simulink model "power_filter"  (R2023b)
settings: Solver=VariableStepAuto  StartTime=0.0  StopTime=.5  RelTol=1e-3
undefined symbols (not defined in the file): T_s, u_gN, w0_pll, w_g
settings Model: Creator=maatt  LastModifiedBy=patet
settings DataIOCC: ReturnWorkspaceOutputs=off

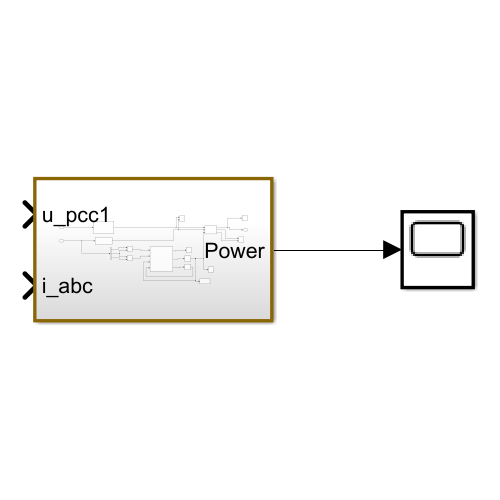
[thumbnail: Simulink's stored preview of the top-level diagram]
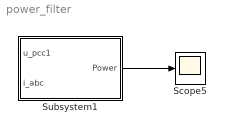
== system power_filter ==
  Scope5 : Scope
  Subsystem1 : Subsystem
  wires:
  Subsystem1/1(Power) -> Scope5/1

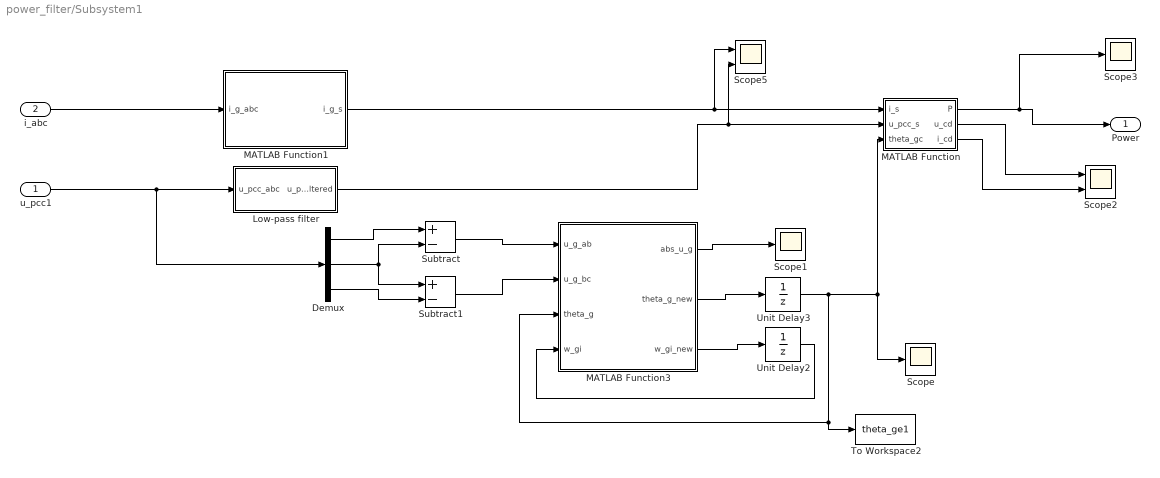
== system power_filter/Subsystem1 ==
  u_pcc1 : Inport
  i_abc : Inport  Port=2
  Demux : Demux  Outputs=3
  Low-pass filter : Subsystem
  MATLAB Function : MATLAB Function  TreatAsAtomicUnit=on
  MATLAB Function1 : MATLAB Function  TreatAsAtomicUnit=on
  MATLAB Function3 : MATLAB Function  TreatAsAtomicUnit=on
  Scope : Scope
  Scope1 : Scope
  Scope2 : Scope  NumInputPorts=2
  Scope3 : Scope
  Scope5 : Scope  NumInputPorts=2
  Subtract : Sum  Inputs=+-
  Subtract1 : Sum  Inputs=+-
  To Workspace2 : ToWorkspace  VariableName=theta_ge1  SaveFormat=Timeseries  SampleTime=-1
  Unit Delay2 : UnitDelay  InitialCondition=w_g  SampleTime=-1  HasFrameUpgradeWarning=on
  Unit Delay3 : UnitDelay  SampleTime=-1  HasFrameUpgradeWarning=on
  Power : Outport
  wires:
  MATLAB Function/1(P) -> Scope3/1, Power/1
  i_abc/1 -> MATLAB Function1/1(i_g_abc)
  Low-pass filter/1(u_pcc_s_filtered) -> Scope5/2, MATLAB Function/2(u_pcc_s)
  Unit Delay2/1 -> MATLAB Function3/4(w_gi)
  MATLAB Function3/2(theta_g_new) -> Unit Delay3/1
  Unit Delay3/1 -> Scope/1, MATLAB Function/3(theta_gc), To Workspace2/1, MATLAB Function3/3(theta_g)
  MATLAB Function3/3(w_gi_new) -> Unit Delay2/1
  u_pcc1/1 -> Demux/1, Low-pass filter/1(u_pcc_abc)
  MATLAB Function3/1(abs_u_g) -> Scope1/1
  Demux/3 -> Subtract1/2
  Subtract/1 -> MATLAB Function3/1(u_g_ab)
  Demux/1 -> Subtract/1
  Demux/2 -> Subtract/2, Subtract1/1
  Subtract1/1 -> MATLAB Function3/2(u_g_bc)
  MATLAB Function/2(u_cd) -> Scope2/1
  MATLAB Function/3(i_cd) -> Scope2/2
  MATLAB Function1/1(i_g_s) -> Scope5/1, MATLAB Function/1(i_s)

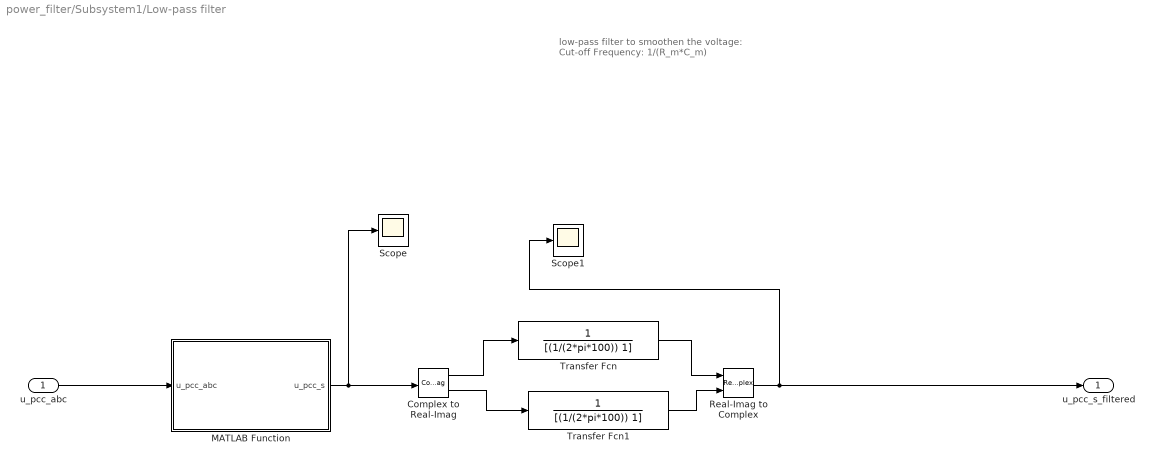
== system power_filter/Subsystem1/Low-pass filter ==
  note: low-pass filter to smoothen the voltage:
      | Cut-off Frequency: 1/(R_m*C_m)
  u_pcc_abc : Inport
  Complex to Real-Imag : ComplexToRealImag
  MATLAB Function : MATLAB Function  TreatAsAtomicUnit=on
  Real-Imag to Complex : RealImagToComplex
  Scope : Scope
  Scope1 : Scope
  Transfer Fcn : TransferFcn  Denominator=[(1/(2*pi*100)) 1]
  Transfer Fcn1 : TransferFcn  Denominator=[(1/(2*pi*100)) 1]
  u_pcc_s_filtered : Outport
  wires:
  Complex to Real-Imag/2 -> Transfer Fcn1/1
  Transfer Fcn/1 -> Real-Imag to Complex/1
  u_pcc_abc/1 -> MATLAB Function/1(u_pcc_abc)
  MATLAB Function/1(u_pcc_s) -> Scope/1, Complex to Real-Imag/1
  Complex to Real-Imag/1 -> Transfer Fcn/1
  Real-Imag to Complex/1 -> Scope1/1, u_pcc_s_filtered/1
  Transfer Fcn1/1 -> Real-Imag to Complex/2

== matlab function power_filter/Subsystem1/MATLAB Function1 ==
  data: i_g_abc input; i_g_s output
function i_g_s  = abc2s(i_g_abc)

% Space Vector Transformation of converter and pcc voltage
i_g_s = 2/3*(i_g_abc(1) + i_g_abc(2)*exp(1j*2*pi/3) + i_g_abc(3)*exp(1j*4*pi/3));

== matlab function power_filter/Subsystem1/MATLAB Function3 ==
  data: abs_u_g output; u_g_ab input size=1; u_g_bc input size=1; theta_g input; w_gi input; u_gN parameter; w0_pll parameter; theta_g_new output; w_gi_new output; T_s parameter
function [abs_u_g, theta_g_new, w_gi_new] = pll(u_g_ab, u_g_bc, theta_g, w_gi, u_gN, w0_pll, T_s)
% Parameters 
% (Tuning of the PLL is analogous to that of the DC-voltage controller.)
zeta = 1;   % Damping ratio
k_p = 2*zeta*w0_pll/u_gN; 
k_i = w0_pll^2/u_gN;

% Space-vector transformation from line-to-line components
u_a = (2*u_g_ab+u_g_bc)/3;
u_b = (-u_g_ab+u_g_bc)/3;
u_c = (-u_g_ab-2*u_g_bc)/3;
u_gs = 2/3*(u_a + u_b*exp(1j*2*pi/3) + u_c*exp(1j*4*pi/3));


% Coordinate transformation to the "estimated" grid coordinates
u_g = u_gs*exp(-1i*theta_g);

% Error signal, which is drive to zero by the PLL
u_gq = imag(u_g);

w_g = k_p*u_gq + w_gi;

% Update the integral state
w_gi_new = w_gi + T_s*k_i*u_gq;

% Update the grid-voltage angle
theta_g_new = theta_g + T_s*w_g;
while(theta_g_new > pi)
    theta_g_new = theta_g_new - 2*pi;
end
while(theta_g_new < -pi)
    theta_g_new = theta_g_new + 2*pi;
end

% Absolute value of the grid-voltage vector
abs_u_g = abs(u_g);

== matlab function power_filter/Subsystem1/Low-pass filter/MATLAB Function ==
  data: u_pcc_abc input; u_pcc_s output
function u_pcc_s  = abc2s(u_pcc_abc)

% Space Vector Transformation of converter and pcc voltage
u_pcc_s = 2/3*(u_pcc_abc(1) + u_pcc_abc(2)*exp(1j*2*pi/3) + u_pcc_abc(3)*exp(1j*4*pi/3));

== matlab function power_filter/Subsystem1/MATLAB Function ==
  data: i_s input; u_pcc_s input; P output; theta_gc input; u_cd output; i_cd output
function [P,u_cd,i_cd] = fcn(i_s, u_pcc_s, theta_gc)
% Reference in stator coordinates
   % Compensation for discrete-time delays
u_cd = (u_pcc_s.*exp(-1j*theta_gc));
i_cd = (i_s.*exp(-1j*theta_gc));
P = 3/2*real((u_cd)*conj(i_cd));
